simulink model "unitdelay"  (Simulink 6.6)
settings: Solver=FixedStepDiscrete  StartTime=0.0  StopTime=10.0  FixedStep=1  RelTol=1e-3
settings Model: Creator=ksmyth  LastModifiedBy=ksmyth

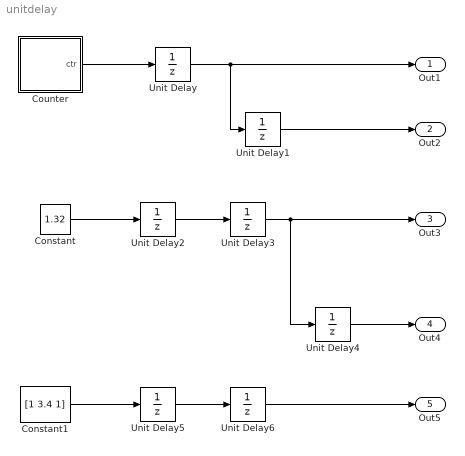
== system unitdelay ==
  Constant : Constant  Value=1.32
  Constant1 : Constant  Value=[1 3.4 1]
  Counter : Stateflow chart
  Unit Delay : UnitDelay
  Unit Delay1 : UnitDelay
  Unit Delay2 : UnitDelay  X0=4
  Unit Delay3 : UnitDelay  X0=2.341
  Unit Delay4 : UnitDelay
  Unit Delay5 : UnitDelay  X0=[0 1 0]
  Unit Delay6 : UnitDelay  X0=[2 3 4]
  Out1 : Outport
  Out2 : Outport  Port=2
  Out3 : Outport  Port=3
  Out4 : Outport  Port=4
  Out5 : Outport  Port=5
  wires:
  Counter/1(ctr) -> Unit Delay/1
  Unit Delay/1 -> Out1/1, Unit Delay1/1
  Unit Delay1/1 -> Out2/1
  Constant/1 -> Unit Delay2/1
  Unit Delay2/1 -> Unit Delay3/1
  Unit Delay3/1 -> Out3/1, Unit Delay4/1
  Unit Delay4/1 -> Out4/1
  Constant1/1 -> Unit Delay5/1
  Unit Delay5/1 -> Unit Delay6/1
  Unit Delay6/1 -> Out5/1

== stateflow chart Counter ==
  state s1
  (default) -> s1
  s1 -> s1 [order 1] : [ctr < 4] / ctr = ctr+1;
  s1 -> s1 [order 2] : [ctr >= 4] / ctr = 0;
  data: ctr output double =1
